simulink model "ee580_final_project"  (R2020b)
settings: Solver=VariableStepAuto  StartTime=0.0  StopTime=10.0  RelTol=1e-3
values from neighbouring files (symbols this model uses):
  Aol = eye(4) + Ac*Ts    [KF_TEST_FPGA.m]    (also in kalman_filter_practice.m = sys_d.A)
  Bol = Bc*Ts    [KF_TEST_FPGA.m]    (also in kalman_filter_practice.m = sys_d.B)
  Col = Cc    [KF_TEST_FPGA.m]    (also in kalman_filter_practice.m = sys_d.C)
  L = 3e-3    (= 0.003)    [KF_TEST_FPGA.m]
undefined symbols (not defined in the file or in its folder): Discrete, Time
libraries: powerlib x23, simulink x5, powerlib_meascontrol x5, re_lib x2, ctrlSharedLib x1
settings Model: Creator=mcapuano  LastModifiedBy=mcapuano

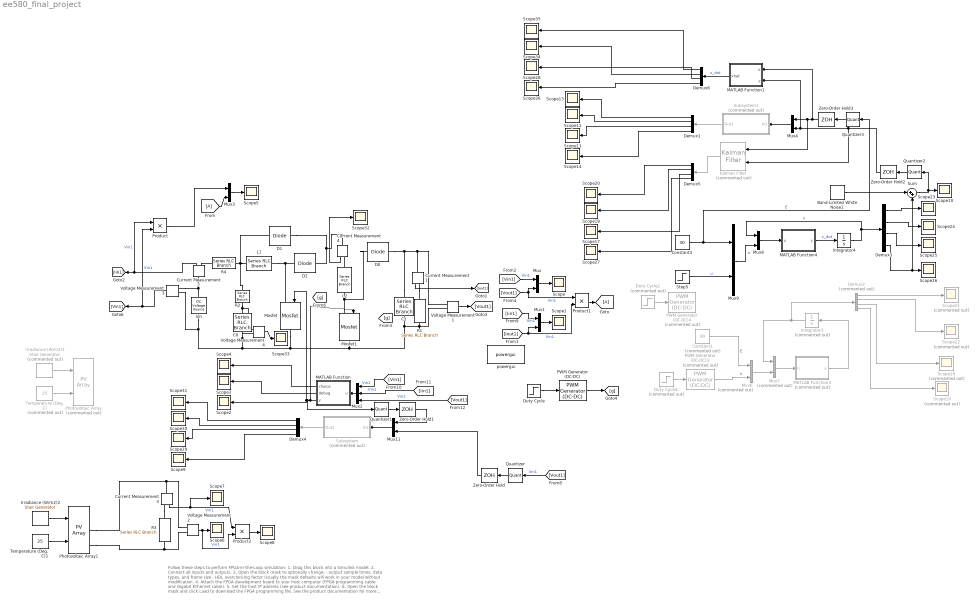
== system ee580_final_project ==
  note: Follow these steps to perform FPGA-in-the-Loop simulation:
      |
      | 1. Drag this block into a Simulink model.
      | 2. Connect all inputs and outputs.
      | 3. Open the block mask to optionally change:
      |     - output sample times, data types, and frame size
      |     - HDL overclocking factor
      |     Usually the mask defaults will work in your model without modification.
      | 4. Attach the FPGA development board to your host computer (FPGA
      |     programming cable and Gigabit Ethernet cable).
      | 5. Set the host IP address (see product documentation).
      | 6. Open the block mask and click Load to download the FPGA programming file.
      |
      | See the product documentation for more detailed instructions and
      | troubleshooting tips.
  Band-Limited White Noise1 : simulink/Sources/Band-Limited White Noise  Cov=[0.000001]  Ts=15e-6  seed=[23341]
  C0 : powerlib/Elements/Series RLC Branch  LConnTagsString=__new0  RConnTagsString=__new0  BranchType=C  Resistance=1e-4  Inductance=200e-6  SetiL0=off  InitialCurrent=0  Capacitance=260e-6  Setx0=on  InitialVoltage=0  Measurements=None
  C1 : powerlib/Elements/Series RLC Branch  LConnTagsString=__new0  RConnTagsString=__new0  BranchType=C  Resistance=1e-4  Inductance=200e-6  SetiL0=off  InitialCurrent=0  Capacitance=260e-6  Setx0=on  InitialVoltage=0  Measurements=None
  Constant1 : Constant  Commented=on  Value=30
  Constant3 : Constant  Value=30
  Current Measurement{1..4} (4 alike) : powerlib/Measurements/Current Measurement  PhasorSimulation=off  OutputType=Complex  PSBequivalent=0
  D0 : powerlib/Power Electronics/Diode  Ron=1e-3  Lon=0  Vf=0  IC=0  UseSnubber=off  Rs=inf  Cs=inf  Measurements=off
  D1 : powerlib/Power Electronics/Diode  Ron=1e-3  Lon=0  Vf=0  IC=0  UseSnubber=off  Rs=inf  Cs=inf  Measurements=off
  D2 : powerlib/Power Electronics/Diode  Ron=1e-3  Lon=0  Vf=0  IC=0  UseSnubber=off  Rs=inf  Cs=inf  Measurements=off
  Demux{1,3..6} (5 alike) : Demux
  Demux2 : Demux  Commented=on
  Duty Cycle : Step  Time=0.5  Before=0.5  After=0.5  SampleTime=0
  Duty Cycle1 : Step  Commented=on  Time=0.5  Before=0.5  After=0.5  SampleTime=0
  Duty Cycle2 : Step  Commented=on  Time=0.5  Before=0.5  After=0.5  SampleTime=0
  Integrator3 : Integrator  Commented=on  InitialCondition=[0 0 0 0]
  Integrator4 : Integrator  InitialCondition=zeros(4,1)
  Irradiance (W/m2)1 : powerlib_meascontrol/Pulse & Signal Generators/Stair Generator  Commented=on  t=[0, 0.5, 1, 1.5, 2]  e=[0.5, 0.7, 0.8, 0.6, 0.2]*1000  Ts=15e-6
  Irradiance (W/m2)2 : powerlib_meascontrol/Pulse & Signal Generators/Stair Generator  t=[0, 0.5, 1, 1.5, 2]  e=[0.5,0.7, 0.8, 0.6, 0.2]*1000  Ts=0.0001
  Kalman Filter : ctrlSharedLib/Kalman Filter  Commented=on  TimeDomain=Discrete-Time  UseCurrentEstimator=on  ModelSource=Individual A, B, C, D matrices  ModelSourceVariable=ss(0.95,1,1,0,1)  A=Aol  B=Bol  C=Col  D=0  NumberOfStates=1  NumberOfInputs=1  NumberOfOutputs=1  InitialEstimateSource=Dialog  X0=0  P0=10  UseK=off  UseGH=off  NumberOfProcessNoiseInputs=1  G=1  TimeInvariantG=on  H=0  TimeInvariantH=on  Q=0.00005  TimeInvariantQ=on  R=100  TimeInvariantR=on  N=0  TimeInvariantN=on  AddInputPort=on  AddEnablePort=off  OutputEstimatedY=off  OutputP=off  Ts=-1
  L1 : powerlib/Elements/Series RLC Branch  LConnTagsString=__new0  RConnTagsString=__new0  BranchType=L  Resistance=1e-4  Inductance=3e-3  SetiL0=on  InitialCurrent=0  Capacitance=30e-6  Setx0=off  InitialVoltage=150  Measurements=None
  L2 : powerlib/Elements/Series RLC Branch  LConnTagsString=__new0  RConnTagsString=__new0  BranchType=L  Resistance=1e-4  Inductance=3e-3  SetiL0=on  InitialCurrent=0  Capacitance=30e-6  Setx0=off  InitialVoltage=150  Measurements=None
  MATLAB Function : MATLAB Function  TreatAsAtomicUnit=on  SystemSampleTime=15e-6
  MATLAB Function1 : MATLAB Function  TreatAsAtomicUnit=on  SystemSampleTime=15e-6
  MATLAB Function3 : MATLAB Function  Commented=on  TreatAsAtomicUnit=on
  MATLAB Function4 : MATLAB Function  TreatAsAtomicUnit=on
  Mosfet : powerlib/Power Electronics/Mosfet  Ron=1e-3  Lon=0  Rd=1e-3  Vfd=0  IC=0  Rs=1e6  Cs=inf  Measurements=off
  Mosfet1 : powerlib/Power Electronics/Mosfet  Ron=1e-3  Lon=0  Rd=1e-3  Vfd=0  IC=0  Rs=1e6  Cs=inf  Measurements=off
  Mux{,1,3..4,8..9,11} (7 alike) : Mux  Inputs=2
  Mux2 : Mux  Inputs=3
  Mux6 : Mux  Commented=on  Inputs=2
  Mux7 : Mux  Commented=on  Inputs=2
  PWM Generator (DC-DC) : powerlib_meascontrol/Pulse & Signal Generators/PWM Generator (DC-DC)  Fsw=66.67e3  Ts=0
  PWM Generator (DC-DC)3 : powerlib_meascontrol/Pulse & Signal Generators/PWM Generator (DC-DC)  Commented=on  Fsw=66.67e3  Ts=0
  PWM Generator (DC-DC)4 : powerlib_meascontrol/Pulse & Signal Generators/PWM Generator (DC-DC)  Commented=on  Fsw=66.67e3  Ts=0
  Photovoltaic Array : re_lib/Solar/PV Array  Commented=on  Npar=1  Nser=1  PlotType=one module @ 25 deg.C & specified irradiances  S_vec=[800]  Temp_C_vec=[ 50 ]  ModuleName=Kyocera Solar KC200GT  PlotWhenSelected=off  Pm=200.143  Ncell=54  Voc=32.9  Isc=8.21  Vm=26.3  Im=7.61  beta_Voc_pc=-0.355  alpha_Isc_pc=0.06  beta_Voc=-0.11679  alpha_Isc=0.004926  IL=8.2288  I0=2.3234e-10  nI=0.97734  Rsh=150.6844  Rs=0.34484  RobustModel=off  RobustCellTemperature=313.3991  BAL=on  Tc=1e-6  Tfilter=5e-5
      settings: AttributesFormatString=|
      | %<ModuleName>
      | %<Nser>-module string
      | %<Npar> parallel strings
  Photovoltaic Array1 : re_lib/Solar/PV Array  Npar=1  Nser=1  PlotType=one module @ 25 deg.C & specified irradiances  S_vec=[800]  Temp_C_vec=[ 50 ]  ModuleName=Kyocera Solar KC200GT  PlotWhenSelected=off  Pm=200.143  Ncell=54  Voc=32.9  Isc=8.21  Vm=26.3  Im=7.61  beta_Voc_pc=-0.355  alpha_Isc_pc=0.06  beta_Voc=-0.11679  alpha_Isc=0.004926  IL=8.2288  I0=2.3234e-10  nI=0.97734  Rsh=150.6844  Rs=0.34484  RobustModel=off  RobustCellTemperature=313.3991  BAL=on  Tc=1e-6  Tfilter=5e-5
      settings: AttributesFormatString=|
      | %<ModuleName>
      | %<Nser>-module string
      | %<Npar> parallel strings
  Product : Product
  Product1 : Product
  Product2 : Product
  Quantizer{,1..3} (4 alike) : Quantizer  QuantizationInterval=15e-6
  R1 : powerlib/Elements/Series RLC Branch  LConnTagsString=__new0  RConnTagsString=__new0  BranchType=R  Resistance=100  Inductance=200e-6  SetiL0=off  InitialCurrent=0  Capacitance=400e-6  Setx0=off  InitialVoltage=0  Measurements=None
  R2 : powerlib/Elements/Series RLC Branch  LConnTagsString=__new0  RConnTagsString=__new0  BranchType=R  Resistance=1e-6  Inductance=200e-6  SetiL0=off  InitialCurrent=0  Capacitance=400e-6  Setx0=off  InitialVoltage=0  Measurements=None
  R3 : powerlib/Elements/Series RLC Branch  LConnTagsString=__new0  RConnTagsString=__new0  BranchType=R  Resistance=1  Inductance=200e-6  SetiL0=off  InitialCurrent=0  Capacitance=400e-6  Setx0=off  InitialVoltage=0  Measurements=None
  R4 : powerlib/Elements/Series RLC Branch  LConnTagsString=__new0  RConnTagsString=__new0  BranchType=R  Resistance=1  Inductance=200e-6  SetiL0=off  InitialCurrent=0  Capacitance=400e-6  Setx0=off  InitialVoltage=0  Measurements=None
  Scope{,1..14,17..18,20,23..36} (32 alike) : Scope
  Scope{16,19,21..22} (4 alike) : Scope  Commented=on
  Step5 : Step  Time=.5  Before=0.5  After=.5  SampleTime=0
  Subsystem : Subsystem  Commented=on
  Subsystem1 : Subsystem  Commented=on
  Sum : Sum  Inputs=|++
  Temperature (Deg. C) : Constant  Commented=on  Value=25
  Temperature (Deg. C)1 : Constant  Value=25
  Vin : powerlib/Electrical Sources/DC Voltage Source  Amplitude=30  Measurements=None
  Voltage Measurement{1..4} (4 alike) : powerlib/Measurements/Voltage Measurement  PhasorSimulation=off  OutputType=Complex  PSBequivalent=0
  Zero-Order Hold{,1..3} (4 alike) : ZeroOrderHold  SampleTime=15e-6
  powergui : powerlib/powergui  Priority=1  SimulationMode=Continuous  SampleTime=50e-6  frequency=60  Iterations=50  frequencyindice=0  Pbase=100e6  ErrMax=1e-4  UnitsV=kV  UnitsW=MW  buscounter=0  FunctionMessages=off  echomessages=off  EnableUseOfTLC=off  CurrentSourceSwitches=off  DisableSnubberDevices=off  DisableRonSwitches=off  DisableVfSwitches=off  DisplayEquations=off  AutomaticDiscreteSolvers=off  SolverType=Tustin/Backward Euler (TBE)  Interpol=off  ExternalGateDelay=off  methode=off  Ts=100  x0status=blocks  SPID=on  SwTol=0  HookPort=off  NonlinearTolerance=1e-4  nMaxIteration=100  ContinueOnMaxIteration=off  RestoreLinks=warning  ResistiveCurrentMeasurement=off  Frange=[0:2:500]  Ylog=off  Xlog=on  ShowGrid=off  save=off  variable=ZData  structure=0  ZoomFFT=off  StartTime=0.0  cycles=1  DisplayStyle=1  fundamental=60  FreqAxis=off  MaxFrequency=1000  frequencyindicesteady=1  RmsSteady=1  display=off
  wires:
  [Iin1] -> Mux2/2  "Vin1"
  Integrator3/1 -> Demux2/1, Mux7/1
  [Vin1] -> Mux2/1  "Vin1"
  [Vout1] -> Quantizer/1  "Vin1"
  Mux6/1 -> Mux7/2
  Irradiance (W/m2)2/1 -> Photovoltaic Array1/1
  Product1/1 -> [A]
  Current Measurement2/1 -> Product/1, [Iin1]  "Vin1"
  Subsystem/1(Out1) -> Demux4/1
  [Iin1] -> Mux1/1  "Vin1"
  [A] -> Mux3/2
  MATLAB Function/1(choice) -> Scope4/1
  Mux2/1 -> MATLAB Function/1(u)
  [Iout1] -> Product1/2, Mux1/2  "Vin1"
  Mux1/1 -> Scope1/1
  PWM Generator (DC-DC)/1 -> [g]
  Duty Cycle/1 -> PWM Generator (DC-DC)/1
  MATLAB Function4/1(y) -> Integrator4/1  "x_dot"
  Temperature (Deg. C)/1 -> Photovoltaic Array/2
  Demux4/2 -> Scope30/1
  Voltage Measurement4/1 -> Scope33/1
  Zero-Order Hold/1 -> Mux11/2
  PWM Generator (DC-DC)3/1 -> Mux6/2  "u"
  Mux11/1 -> Subsystem/1(In1)
  Mux9/1 -> Mux8/2  "u"
  Voltage Measurement1/1 -> [Vout1]
  Demux3/1 -> Scope23/1
  Demux3/3 -> Scope25/1
  Demux3/2 -> Scope24/1
  Constant3/1 -> Quantizer3/1, Mux9/1  "E"
  Mux8/1 -> MATLAB Function4/1(u)
  Demux2/4 -> Scope19/1
  Temperature (Deg. C)1/1 -> Photovoltaic Array1/2
  Mux/1 -> Scope/1
  Product/1 -> Mux3/1
  Demux2/2 -> Scope22/1
  [Vout1] -> Mux/2, Product1/1  "Vin1"
  Mux3/1 -> Scope5/1
  Mux7/1 -> MATLAB Function3/1(u)
  MATLAB Function3/1(y) -> Integrator3/1
  MATLAB Function/2(debug) -> Scope3/1
  Duty Cycle1/1 -> PWM Generator (DC-DC)3/1
  Irradiance (W/m2)1/1 -> Photovoltaic Array/1
  Voltage Measurement2/1 -> Product2/2, Scope6/1  "Vin1"
  Demux2/3 -> Scope16/1
  Product2/1 -> Scope8/1
  Demux3/4 -> Sum/2, Scope26/1
  Voltage Measurement3/1 -> Product/2, [Vin1]  "Vin1"
  Duty Cycle2/1 -> PWM Generator (DC-DC)4/1
  Quantizer1/1 -> Zero-Order Hold1/1
  Current Measurement3/1 -> Product2/1, Scope7/1  "Vin1"
  Integrator4/1 -> Mux8/1, Demux3/1  "x"
  Quantizer/1 -> Zero-Order Hold/1
  MATLAB Function/3(y) -> Mosfet1/1, Mosfet/1, Scope2/1, Quantizer1/1
  Demux4/1 -> Scope31/1
  [Vout1] -> Mux2/3  "Vin1"
  Constant1/1 -> Mux6/1  "E"
  Demux2/1 -> Scope21/1
  Current Measurement1/1 -> [Iout1]
  Current Measurement4/1 -> Scope32/1
  [Vin1] -> Mux/1  "Vin1"
  Demux4/3 -> Scope29/1
  Demux4/4 -> Scope9/1
  Step5/1 -> Mux9/2  "u"
  Zero-Order Hold1/1 -> Mux11/1
  Mux4/1 -> Subsystem1/1(In1)
  Quantizer2/1 -> Zero-Order Hold2/1
  Zero-Order Hold2/1 -> Kalman Filter/2, MATLAB Function1/2(y), Mux4/2
  Demux1/1 -> Scope13/1
  Demux1/2 -> Scope12/1
  Demux1/3 -> Scope11/1
  Subsystem1/1(Out1) -> Demux1/1
  Quantizer3/1 -> Zero-Order Hold3/1
  Zero-Order Hold3/1 -> MATLAB Function1/1(u), Kalman Filter/1, Mux4/1
  Band-Limited White Noise1/1 -> Sum/1
  Sum/1 -> Scope10/1, Quantizer2/1
  Demux1/4 -> Scope14/1
  Kalman Filter/1 -> Demux5/1
  Demux5/4 -> Scope27/1
  Demux5/3 -> Scope17/1
  Demux5/2 -> Scope18/1
  Demux5/1 -> Scope20/1
  MATLAB Function1/1(xhat) -> Demux6/1  "x_dot"
  Demux6/1 -> Scope35/1
  Demux6/2 -> Scope34/1
  Demux6/3 -> Scope28/1
  Demux6/4 -> Scope36/1
  connections:
  C1/LConn1 -- Current Measurement1/LConn1 -- Voltage Measurement1/LConn1 -- D0/RConn1
  L2/RConn1 -- D0/LConn1 -- Mosfet1/LConn1
  C0/RConn1 -- Voltage Measurement4/LConn2 -- Vin/LConn1 -- Voltage Measurement3/LConn2 -- C1/RConn1 -- Voltage Measurement1/LConn2 -- R1/RConn1 -- Mosfet1/RConn1 -- Mosfet/RConn1
  D1/LConn1 -- R4/RConn1 -- L1/LConn1 -- R2/LConn1
  D2/RConn1 -- D1/RConn1 -- Current Measurement4/LConn1
  C0/LConn1 -- R2/RConn1 -- Voltage Measurement4/LConn1
  R3/RConn1 -- Photovoltaic Array1/RConn2 -- Voltage Measurement2/LConn2
  Voltage Measurement2/LConn1 -- Photovoltaic Array1/RConn1 -- Current Measurement3/LConn1
  Voltage Measurement3/LConn1 -- Vin/RConn1 -- Current Measurement2/LConn1
  Mosfet/LConn1 -- L1/RConn1 -- D2/LConn1
  L2/LConn1 -- Current Measurement4/RConn1
  Current Measurement3/RConn1 -- R3/LConn1
  Current Measurement1/RConn1 -- R1/LConn1
  R4/LConn1 -- Current Measurement2/RConn1

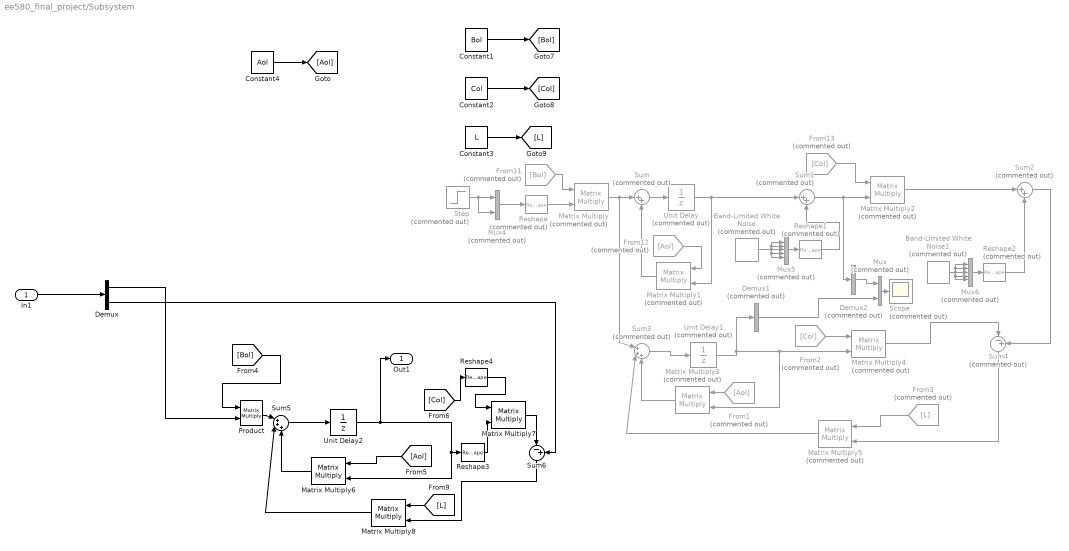
== system ee580_final_project/Subsystem ==
  In1 : Inport
  Band-Limited White Noise : simulink/Sources/Band-Limited White Noise  Commented=on  Cov=[0.1]  Ts=.05  seed=[23341]
  Band-Limited White Noise1 : simulink/Sources/Band-Limited White Noise  Commented=on  Cov=[0.1]  Ts=.05  seed=[23341]
  Constant1 : Constant  Value=Bol
  Constant2 : Constant  Value=Col
  Constant3 : Constant  Value=L
  Constant4 : Constant  Value=Aol
  Demux : Demux  Outputs=2
  Demux1 : Demux  Commented=on  Outputs=5
  Demux2 : Demux  Commented=on  Outputs=5
  From1 : From  Commented=on  GotoTag=Aol
  From11 : From  Commented=on  GotoTag=Bol
  From12 : From  Commented=on  GotoTag=Aol
  From13 : From  Commented=on  GotoTag=Col
  From2 : From  Commented=on  GotoTag=Col
  From3 : From  Commented=on  GotoTag=L
  Matrix Multiply{,1..5} (6 alike) : Product  Commented=on  Multiplication=Matrix(*)
  Matrix Multiply6 : Product  Multiplication=Matrix(*)
  Matrix Multiply7 : Product  Multiplication=Matrix(*)
  Matrix Multiply8 : Product  Multiplication=Matrix(*)
  Mux : Mux  Commented=on  Inputs=2
  Mux4 : Mux  Commented=on  Inputs=2
  Mux5 : Mux  Commented=on  Inputs=5
  Mux6 : Mux  Commented=on  Inputs=5
  Product : Product  Multiplication=Matrix(*)
  Reshape : Reshape  Commented=on  OutputDimensionality=Customize  OutputDimensions=[2,1]
  Reshape1 : Reshape  Commented=on  OutputDimensionality=Customize  OutputDimensions=[5,1]
  Reshape2 : Reshape  Commented=on  OutputDimensionality=Customize  OutputDimensions=[5,1]
  Reshape3 : Reshape  OutputDimensionality=Customize  OutputDimensions=[4,1]
  Reshape4 : Reshape  OutputDimensionality=Customize  OutputDimensions=[1,4]
  Scope : Scope  Commented=on
  Step : Step  Commented=on  SampleTime=0
  Sum : Sum  Commented=on  Inputs=|++
  Sum1 : Sum  Commented=on  Inputs=|++
  Sum2 : Sum  Commented=on  Inputs=|++
  Sum3 : Sum  Commented=on  Inputs=|+++
  Sum4 : Sum  Commented=on  Inputs=|-+
  Sum5 : Sum  Inputs=|+++
  Sum6 : Sum  Inputs=|-+
  Unit Delay : UnitDelay  Commented=on  SampleTime=-1  HasFrameUpgradeWarning=on
  Unit Delay1 : UnitDelay  Commented=on  SampleTime=-1  HasFrameUpgradeWarning=on
  Unit Delay2 : UnitDelay  SampleTime=-1  HasFrameUpgradeWarning=on
  Out1 : Outport
  wires:
  From1/1 -> Matrix Multiply3/1
  Band-Limited White Noise/1 -> Mux5/2, Mux5/1, Mux5/5, Mux5/4, Mux5/3
  Mux4/1 -> Reshape/1
  Mux/1 -> Scope/1
  Demux2/3 -> Mux/1
  Matrix Multiply4/1 -> Sum4/1
  From3/1 -> Matrix Multiply5/1
  From12/1 -> Matrix Multiply1/1
  Reshape1/1 -> Sum1/2
  Matrix Multiply5/1 -> Sum3/2
  Matrix Multiply3/1 -> Sum3/3
  From2/1 -> Matrix Multiply4/1
  Sum1/1 -> Demux2/1, Matrix Multiply2/2
  Sum4/1 -> Matrix Multiply5/2
  Unit Delay1/1 -> Demux1/1, Matrix Multiply3/2, Matrix Multiply4/2
  Band-Limited White Noise1/1 -> Mux6/2, Mux6/1, Mux6/5, Mux6/4, Mux6/3
  Constant3/1 -> [L]
  Sum2/1 -> Sum4/2
  Reshape2/1 -> Sum2/2
  Reshape/1 -> Matrix Multiply/2
  Demux1/3 -> Mux/2
  Sum3/1 -> Unit Delay1/1
  Constant2/1 -> [Col]
  Sum/1 -> Unit Delay/1
  From11/1 -> Matrix Multiply/1
  Mux6/1 -> Reshape2/1
  Mux5/1 -> Reshape1/1
  From13/1 -> Matrix Multiply2/1
  Matrix Multiply1/1 -> Sum/2
  Matrix Multiply/1 -> Sum3/1, Sum/1
  Unit Delay/1 -> Matrix Multiply1/2, Sum1/1
  Matrix Multiply2/1 -> Sum2/1
  Step/1 -> Mux4/2, Mux4/1
  Constant1/1 -> [Bol]
  In1/1 -> Demux/1
  Demux/2 -> Sum6/2
  Constant4/1 -> [Aol]
  [Bol] -> Product/1
  Product/1 -> Sum5/1
  Sum5/1 -> Unit Delay2/1
  [Aol] -> Matrix Multiply6/1
  Unit Delay2/1 -> Out1/1, Reshape3/1, Matrix Multiply6/2
  Matrix Multiply6/1 -> Sum5/3
  Matrix Multiply7/1 -> Sum6/1
  [L] -> Matrix Multiply8/1
  Sum6/1 -> Matrix Multiply8/2
  Matrix Multiply8/1 -> Sum5/2
  Demux/1 -> Product/2
  Reshape3/1 -> Matrix Multiply7/2
  [Col] -> Reshape4/1
  Reshape4/1 -> Matrix Multiply7/1

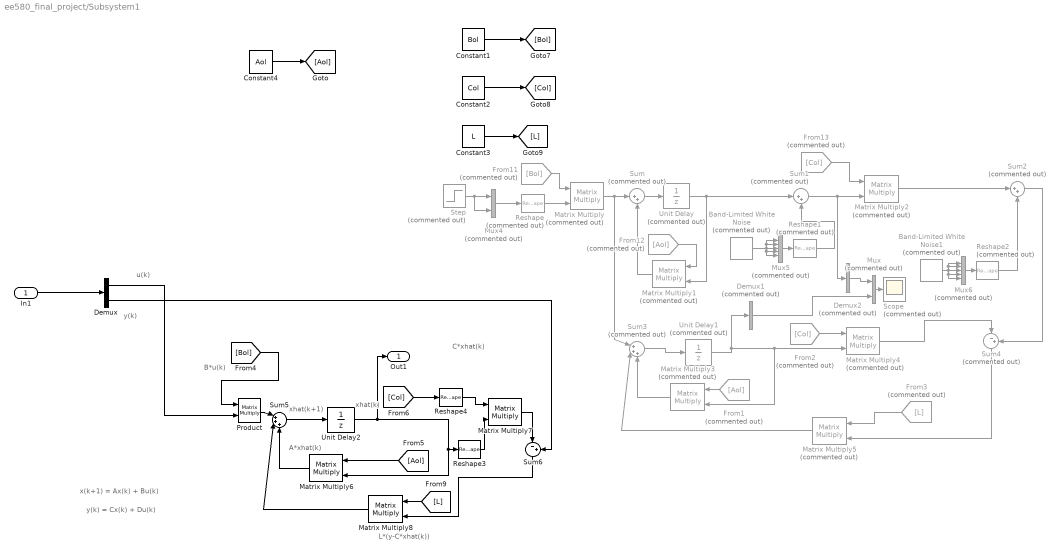
== system ee580_final_project/Subsystem1 ==
  note: y(k)
  note: u(k)
  note: y(k) = Cx(k) + Du(k)
  note: x(k+1) = Ax(k) + Bu(k)
  note: C*xhat(k)
  note: L*(y-C*xhat(k))
  note: B*u(k)
  note: A*xhat(k)
  note: xhat(k)
  note: xhat(k+1)
  In1 : Inport
  Band-Limited White Noise : simulink/Sources/Band-Limited White Noise  Commented=on  Cov=[0.1]  Ts=.05  seed=[23341]
  Band-Limited White Noise1 : simulink/Sources/Band-Limited White Noise  Commented=on  Cov=[0.1]  Ts=.05  seed=[23341]
  Constant1 : Constant  Value=Bol
  Constant2 : Constant  Value=Col
  Constant3 : Constant  Value=L
  Constant4 : Constant  Value=Aol
  Demux : Demux  Outputs=2
  Demux1 : Demux  Commented=on  Outputs=5
  Demux2 : Demux  Commented=on  Outputs=5
  From1 : From  Commented=on  GotoTag=Aol
  From11 : From  Commented=on  GotoTag=Bol
  From12 : From  Commented=on  GotoTag=Aol
  From13 : From  Commented=on  GotoTag=Col
  From2 : From  Commented=on  GotoTag=Col
  From3 : From  Commented=on  GotoTag=L
  Matrix Multiply{,1..5} (6 alike) : Product  Commented=on  Multiplication=Matrix(*)
  Matrix Multiply6 : Product  Multiplication=Matrix(*)
  Matrix Multiply7 : Product  Multiplication=Matrix(*)
  Matrix Multiply8 : Product  Multiplication=Matrix(*)
  Mux : Mux  Commented=on  Inputs=2
  Mux4 : Mux  Commented=on  Inputs=2
  Mux5 : Mux  Commented=on  Inputs=5
  Mux6 : Mux  Commented=on  Inputs=5
  Product : Product  Multiplication=Matrix(*)
  Reshape : Reshape  Commented=on  OutputDimensionality=Customize  OutputDimensions=[2,1]
  Reshape1 : Reshape  Commented=on  OutputDimensionality=Customize  OutputDimensions=[5,1]
  Reshape2 : Reshape  Commented=on  OutputDimensionality=Customize  OutputDimensions=[5,1]
  Reshape3 : Reshape  OutputDimensionality=Customize  OutputDimensions=[4,1]
  Reshape4 : Reshape  OutputDimensionality=Customize  OutputDimensions=[1,4]
  Scope : Scope  Commented=on
  Step : Step  Commented=on  SampleTime=0
  Sum : Sum  Commented=on  Inputs=|++
  Sum1 : Sum  Commented=on  Inputs=|++
  Sum2 : Sum  Commented=on  Inputs=|++
  Sum3 : Sum  Commented=on  Inputs=|+++
  Sum4 : Sum  Commented=on  Inputs=|-+
  Sum5 : Sum  Inputs=|+++
  Sum6 : Sum  Inputs=|-+
  Unit Delay : UnitDelay  Commented=on  SampleTime=-1  HasFrameUpgradeWarning=on
  Unit Delay1 : UnitDelay  Commented=on  SampleTime=-1  HasFrameUpgradeWarning=on
  Unit Delay2 : UnitDelay  SampleTime=-1  HasFrameUpgradeWarning=on
  Out1 : Outport
  wires:
  From1/1 -> Matrix Multiply3/1
  Band-Limited White Noise/1 -> Mux5/2, Mux5/1, Mux5/5, Mux5/4, Mux5/3
  Mux4/1 -> Reshape/1
  Mux/1 -> Scope/1
  Demux2/3 -> Mux/1
  Matrix Multiply4/1 -> Sum4/1
  From3/1 -> Matrix Multiply5/1
  From12/1 -> Matrix Multiply1/1
  Reshape1/1 -> Sum1/2
  Matrix Multiply5/1 -> Sum3/2
  Matrix Multiply3/1 -> Sum3/3
  From2/1 -> Matrix Multiply4/1
  Sum1/1 -> Demux2/1, Matrix Multiply2/2
  Sum4/1 -> Matrix Multiply5/2
  Unit Delay1/1 -> Demux1/1, Matrix Multiply3/2, Matrix Multiply4/2
  Band-Limited White Noise1/1 -> Mux6/2, Mux6/1, Mux6/5, Mux6/4, Mux6/3
  Constant3/1 -> [L]
  Sum2/1 -> Sum4/2
  Reshape2/1 -> Sum2/2
  Reshape/1 -> Matrix Multiply/2
  Demux1/3 -> Mux/2
  Sum3/1 -> Unit Delay1/1
  Constant2/1 -> [Col]
  Sum/1 -> Unit Delay/1
  From11/1 -> Matrix Multiply/1
  Mux6/1 -> Reshape2/1
  Mux5/1 -> Reshape1/1
  From13/1 -> Matrix Multiply2/1
  Matrix Multiply1/1 -> Sum/2
  Matrix Multiply/1 -> Sum3/1, Sum/1
  Unit Delay/1 -> Matrix Multiply1/2, Sum1/1
  Matrix Multiply2/1 -> Sum2/1
  Step/1 -> Mux4/2, Mux4/1
  Constant1/1 -> [Bol]
  In1/1 -> Demux/1
  Demux/2 -> Sum6/2
  Constant4/1 -> [Aol]
  [Bol] -> Product/1
  Product/1 -> Sum5/1
  Sum5/1 -> Unit Delay2/1
  [Aol] -> Matrix Multiply6/1
  Unit Delay2/1 -> Out1/1, Reshape3/1, Matrix Multiply6/2
  Matrix Multiply6/1 -> Sum5/3
  Matrix Multiply7/1 -> Sum6/1
  [L] -> Matrix Multiply8/1
  Sum6/1 -> Matrix Multiply8/2
  Matrix Multiply8/1 -> Sum5/2
  Demux/1 -> Product/2
  Reshape3/1 -> Matrix Multiply7/2
  [Col] -> Reshape4/1
  Reshape4/1 -> Matrix Multiply7/1

== matlab function ee580_final_project/MATLAB Function1 ==
  data: u input; xhat output; y input
function xhat  = fcn(u, y)
%Kalman filter design using Small Signal Model of Circuit

%The purpose of this module is to approximate Ipv and Vpv so that a sensor
%is not needed for those variables, it also functions to remove noise and
%could possibly replace the MCP module using its own predictions

%Existing Model assumes Constant Vpv with added series resistor so that
% Ipv = (Vpv - Vcpv)/Rpv
%Also assumes L1 = L2

%Existing state variables: IL1 IL2 Vo Vcpv

%define circuit parameters 

Cpv=260e-6;
Cout=260e-6;
L1=3e-3;
L2=3e-3;
Rout=100;
Rpv = 1;
RL1 = 1;
RL2 = 1;


Vpv = 30;

u_e = .5;

Ts = 15e-6;
% Continuous Time Small Signal State Space
%Aol = [0.943784461257301,-0.0559330122345799,-0.0279395312339836,5.29606701473712e-05;0.00363447688363775,0.996152021590196,-0.00131615408875196,-0.00124644633684318;0.00363447688363775,-0.00135110080726459,0.996186968308708,-0.00124644633684318;5.29606701473712e-05,-1.90030480999995e-05,0.0287831492829427,0.999405251934562];
Ac =[(-1/(Cpv*Rpv)) (-1/(Cpv)) (-u_e/(Cpv)) 0 ;
    (1/(L1+L2) + L2*u_e/(L1*(L1+L2)))  (-RL1/(L1+L2) -RL1*L2*u_e/(L1*(L1+L2)))  (-RL2/(L1+L2) + RL2*u_e/(L1+L2)) (-1/(L1+L2) + u_e/(L1+L2));
    (1/(L1+L2) + L1*u_e/(L2*(L1+L2)))  (-RL1/(L1+L2) + RL1*u_e/(L1+L2)) (-RL2/(L1+L2)-RL2*L1*u_e/(L2*(L1+L2))) (-1/(L1+L2) + u_e/(L1+L2));
    0 0 (1/(Cout) - u_e/(Cout)) (-1/(Rout*Cout))];
Bc = [1/(Cpv*Rpv);
    0;
    0;
    0];
 Cc = [0 0 0 1];
 
 Dc = zeros(size(Cc,1), size(Bc,2));
 
 Aol = eye(4) + Ac*Ts;
 Bol = Bc*Ts;
 Col = Cc;
 Dol = Dc;
 
%Bol = [0.0560566260169120;0.000105941817191590;0.000105941817191590;1.02384484238660e-06];

%Col = [0,0,0,1];

%Dol = 0;
 %Design the Observer System:
 
 %G and H
 G = eye(4); % 4 states, 4 disturbances
 H = [0 0 0 0]; %not including W noise for output
 
 %covar matricies, process q, measurement r -- must be positive numbers
 Qcov = diag(.000001*ones(1,4)); %tweak the numbers to change how it filters noise
 Rcov = diag(10*ones(1,1)); %tweak the numbers to change how it filters noise
 

persistent xhat_t_1; %previous xhat Sample
if isempty(xhat_t_1)
    xhat_t_1 = [.1; .1; .1; .1];
end

persistent P_t_1;
if isempty(P_t_1)
    P_t_1 = [.1 .1 .1 .1;
            .1 .1 .1 .1;
            .1 .1 .1 .1;
            .1 .1 .1 .1];
end


%prediction stage
xhat_pred = Aol*xhat_t_1+Bol*u;
P_pred = Aol*P_t_1*transpose(Aol)+ Qcov;

%update stage
y_update = y - Col*xhat_pred;
S_update = Col*P_pred*transpose(Col) + Rcov;
K_update = P_pred*transpose(Col)*(1/S_update);
xhat_update = xhat_pred + K_update*y_update;
P_update = (eye(4) - K_update*Col)*P_pred;



%update function output and variables
P_t_1 = P_update;
xhat_t_1 = xhat_update;
xhat = xhat_update;

== matlab function ee580_final_project/MATLAB Function ==
  settings: updateMethod=DISCRETE
  data: choice output; debug output; u input; y output
function [choice, debug, y]= fcn(u)
Vpv=u(1);
Ipv=u(2);
Vout=u(3);

%This module contains the MPC-MPPT Control Algorithm

%The MPC module follows the flow chart of Fig. 8 in Referenced Research Paper

%This MATLAB fn block's settings have been changed to have a sampling rate
%of 15uS instead of being continous sample mode


%prevent crazy simulation transients from breaking the algorithm:
if (Ipv > 10)
    Ipv = 1;
end

persistent Vpv_t_1; %previous Vpv Sample
if isempty(Vpv_t_1)
    Vpv_t_1 = 0;
end
persistent Ipv_t_1; %previous Ipv Sample
if isempty(Ipv_t_1)
    Ipv_t_1 = 0;
end
persistent Dpv_t_1; % Iref (output) value from what is now 2 timesteps ago
if isempty(Dpv_t_1)
    Dpv_t_1 = 0;
end
persistent Dpv;  %Previous / Most recent Iref (output) Calc
if isempty(Dpv)
    Dpv = 0;
end

Ts = 15e-6; %sample rate
L = 3e-3; %inductance


delta_V = Vpv - Vpv_t_1;
delta_I = Ipv - Ipv_t_1;
delta_D = Dpv - Dpv_t_1;


%fixed vs adaptive
scale_factor_C = 10; %increase for larger output increments/swings
 Z =.01; %fixed 
%Z = scale_factor_C * abs(delta_I * delta_D); %adaptive

% custom adaptive to fix issues with no change causing 0 step size
 adapZ = scale_factor_C * abs(delta_I * delta_D);
% if(adapZ > .1)
%     Z = .1;
% elseif(adapZ > .001)
%     Z = adapZ;
% else
%     Z = .001;
% end

Ipred_1 = Ipv + 2*(Ts/L) * Vpv; %MPC prediction for switch = 1
Ipred_0 = Ipv + (Ts/(2*L)* (Vpv - Vout)); %MPC prediction for switch = 0 

if delta_V == 0 %Inc. Cond. Algo to determin Iref
    if delta_I == 0 
        Iref = Dpv; choice = 0;
    else
        if delta_I > 0
            Iref = Dpv - Z; choice = 1;
        else
            Iref = Dpv + Z; choice = 2;
        end
    end
else
    if (Ipv + (delta_I/delta_V) * Vpv) == 0
        Iref = Dpv; choice = 3;
    else
        if (Ipv + (delta_I/delta_V) * Vpv) > 0
            Iref = Dpv - Z; choice = 4;
        else
            Iref = Dpv + Z; choice = 5;
        end
    end
end

G1 = abs(Iref - Ipred_1); %Optimize MPC by applying Iref
G0 = abs(Iref - Ipred_0);
if G1 < G0
    y = 1;
else
    y = 0;
end

if (Iref < 0)
    Iref = .001;
end
%test = Ipv + (delta_I/delta_V) * Vpv;
test =  delta_V;
%update static variables here:
Vpv_t_1 = Vpv; %previous Vpv Sample
Ipv_t_1 = Ipv; %previous Ipv Sample
Dpv_t_1 = Dpv; % Iref (output) value from what is now 2 timesteps ago
Dpv = Iref;  %Previous / Most recent Iref (output) Calc

%debug purposes:
debug = Iref;

== matlab function ee580_final_project/MATLAB Function3 ==
  data: u input; y output
function y = fcn(u)

X=u(1:4);
Vpv=u(5);
u=u(6);



% parameters:


Cpv=260e-6;
Co=260e-6;
L1=3e-3;
L2=3e-3;
R=100;
Rpv = 1;

% Compact form
A=[ 0 0 -1/(2*L1) 1/(2*L1) ;
    0 0 -1/(2*L2) 1/(2*L2) ;
    0 1/Co  -1/(R*Co) 0;
    -1/Cpv 0 0 -1/(Rpv*Cpv)];

B=[0 0 1/(2*L1) 1/(2*L1);
    0 0 1/(2*L2) 1/(2*L2);
     0 -1/Co 0 0;
    0 -1/Cpv 0 0 ];
     
     
b=[0; 0; 0; 0];

d=[0; 0; 0; Vpv/(Rpv*Cpv)];

y = A*X+(B*X+b)*u+d;

== matlab function ee580_final_project/MATLAB Function4 ==
  data: u input; y output
function y = fcn(u)

X=u(1:4);
Vpv=u(5);
u=u(6);



% parameters:
%5/10/2021 u_ePDATED


Cpv=260e-6;
Cout=260e-6;
L1=3e-3;
L2=3e-3;
Rout=100;
Rpv = 1;
RL1 = 1;
RL2 = 1;

u_e = .5;

% Compact form
A=[(-1/(Cpv*Rpv)) (-1/(Cpv)) (-u_e/(Cpv)) 0 ;
    (1/(L1+L2) + L2*u_e/(L1*(L1+L2)))  (-RL1/(L1+L2) -RL1*L2*u_e/(L1*(L1+L2)))  (-RL2/(L1+L2) + RL2*u_e/(L1+L2)) (-1/(L1+L2) + u_e/(L1+L2));
    (1/(L1+L2) + L1*u_e/(L2*(L1+L2)))  (-RL1/(L1+L2) + RL1*u_e/(L1+L2)) (-RL2/(L1+L2)-RL2*L1*u_e/(L2*(L1+L2))) (-1/(L1+L2) + u_e/(L1+L2));
    0 0 (1/(Cout) - u_e/(Cout)) (-1/(Rout*Cout))];

%VCpv = (L2*RL1*Rout*Vpv*u_e^2 - 2*L2*RL1*Rout*Vpv*u_e + L1*RL1*RL2*Vpv + L2*RL1*RL2*Vpv + L2*RL1*Rout*Vpv)/(L1*RL1*RL2 + L2*RL1*RL2 + L2*RL1*Rout + L2*RL2*Rpv - L1*Rout*Rpv + L2*Rout*Rpv + L2*RL1*Rout*u_e^2 + L2*RL1*Rpv*u_e^2 - L1*Rout*Rpv*u_e^2 + L2*Rout*Rpv*u_e^2 - 2*L2*RL1*Rout*u_e + L1*RL1*Rpv*u_e + L1*RL2*Rpv*u_e + 2*L1*Rout*Rpv*u_e - 2*L2*Rout*Rpv*u_e);
%IL1 = (Vpv*(L2*RL2 - L1*Rout + L2*Rout + L1*RL2*u_e + 2*L1*Rout*u_e - 2*L2*Rout*u_e - L1*Rout*u_e^2 + L2*Rout*u_e^2))/(L1*RL1*RL2 + L2*RL1*RL2 + L2*RL1*Rout + L2*RL2*Rpv - L1*Rout*Rpv + L2*Rout*Rpv + L2*RL1*Rout*u_e^2 + L2*RL1*Rpv*u_e^2 - L1*Rout*Rpv*u_e^2 + L2*Rout*Rpv*u_e^2 - 2*L2*RL1*Rout*u_e + L1*RL1*Rpv*u_e + L1*RL2*Rpv*u_e + 2*L1*Rout*Rpv*u_e - 2*L2*Rout*Rpv*u_e);
%IL2 = (RL1*Vpv*(L1 + L2*u_e))/(L1*RL1*RL2 + L2*RL1*RL2 + L2*RL1*Rout + L2*RL2*Rpv - L1*Rout*Rpv + L2*Rout*Rpv + L2*RL1*Rout*u_e^2 + L2*RL1*Rpv*u_e^2 - L1*Rout*Rpv*u_e^2 + L2*Rout*Rpv*u_e^2 - 2*L2*RL1*Rout*u_e + L1*RL1*Rpv*u_e + L1*RL2*Rpv*u_e + 2*L1*Rout*Rpv*u_e - 2*L2*Rout*Rpv*u_e);
%VCout = -(RL1*Rout*Vpv*(L1 + L2*u_e)*(u_e - 1))/(L1*RL1*RL2 + L2*RL1*RL2 + L2*RL1*Rout + L2*RL2*Rpv - L1*Rout*Rpv + L2*Rout*Rpv + L2*RL1*Rout*u_e^2 + L2*RL1*Rpv*u_e^2 - L1*Rout*Rpv*u_e^2 + L2*Rout*Rpv*u_e^2 - 2*L2*RL1*Rout*u_e + L1*RL1*Rpv*u_e + L1*RL2*Rpv*u_e + 2*L1*Rout*Rpv*u_e - 2*L2*Rout*Rpv*u_e);

VCpv = (L2*RL1*Rout*Vpv*u_e^2 - 2*L2*RL1*Rout*Vpv*u_e + L1*RL1*RL2*Vpv + L2*RL1*RL2*Vpv + L2*RL1*Rout*Vpv)/(L1*RL1*RL2 + L2*RL1*RL2 + L2*RL1*Rout + L2*RL2*Rpv - L1*Rout*Rpv + L2*Rout*Rpv + L2*RL1*Rout*u_e^2 + L2*RL1*Rpv*u_e^2 - L1*Rout*Rpv*u_e^2 + L2*Rout*Rpv*u_e^2 - 2*L2*RL1*Rout*u_e + L1*RL1*Rpv*u_e + L1*RL2*Rpv*u_e + 2*L1*Rout*Rpv*u_e - 2*L2*Rout*Rpv*u_e);
IL1 = (Vpv*(L2*RL2 - L1*Rout + L2*Rout + L1*RL2*u_e + 2*L1*Rout*u_e - 2*L2*Rout*u_e - L1*Rout*u_e^2 + L2*Rout*u_e^2))/(L1*RL1*RL2 + L2*RL1*RL2 + L2*RL1*Rout + L2*RL2*Rpv - L1*Rout*Rpv + L2*Rout*Rpv + L2*RL1*Rout*u_e^2 + L2*RL1*Rpv*u_e^2 - L1*Rout*Rpv*u_e^2 + L2*Rout*Rpv*u_e^2 - 2*L2*RL1*Rout*u_e + L1*RL1*Rpv*u_e + L1*RL2*Rpv*u_e + 2*L1*Rout*Rpv*u_e - 2*L2*Rout*Rpv*u_e);
IL2 =  (RL1*Vpv*(L1 + L2*u_e))/(L1*RL1*RL2 + L2*RL1*RL2 + L2*RL1*Rout + L2*RL2*Rpv - L1*Rout*Rpv + L2*Rout*Rpv + L2*RL1*Rout*u_e^2 + L2*RL1*Rpv*u_e^2 - L1*Rout*Rpv*u_e^2 + L2*Rout*Rpv*u_e^2 - 2*L2*RL1*Rout*u_e + L1*RL1*Rpv*u_e + L1*RL2*Rpv*u_e + 2*L1*Rout*Rpv*u_e - 2*L2*Rout*Rpv*u_e);
VCout =  -(RL1*Rout*Vpv*(L1 + L2*u_e)*(u_e - 1))/(L1*RL1*RL2 + L2*RL1*RL2 + L2*RL1*Rout + L2*RL2*Rpv - L1*Rout*Rpv + L2*Rout*Rpv + L2*RL1*Rout*u_e^2 + L2*RL1*Rpv*u_e^2 - L1*Rout*Rpv*u_e^2 + L2*Rout*Rpv*u_e^2 - 2*L2*RL1*Rout*u_e + L1*RL1*Rpv*u_e + L1*RL2*Rpv*u_e + 2*L1*Rout*Rpv*u_e - 2*L2*Rout*Rpv*u_e);
 
% B=[ -IL2/Cpv;
%     L2*VCpv/(L1*(L1+L2))-RL1*L2*IL1/(L1*(L1+L2))+RL2*IL2/(L1+L2)+VCout/(L1+L2);
%     L1*VCpv/(L2*(L1+L2))+RL1*IL1/(L1+L2)-RL2*L1*IL2/(L2*(L1+L2))+VCout/(L1+L2);
%      -IL2/Cout];


B = [1/(Cpv*Rpv);
    0;
    0;
    0];

u = Vpv;

y = A*X+B*u;
